simulink model "PhilippePetit"  (R2020b)
settings: Solver=VariableStepAuto  StartTime=0.0  StopTime=10.0  RelTol=1e-3
undefined symbols (not defined in the file or in its folder): den, num_beta, num_x
settings Model: Creator=nicol  LastModifiedBy=nicol

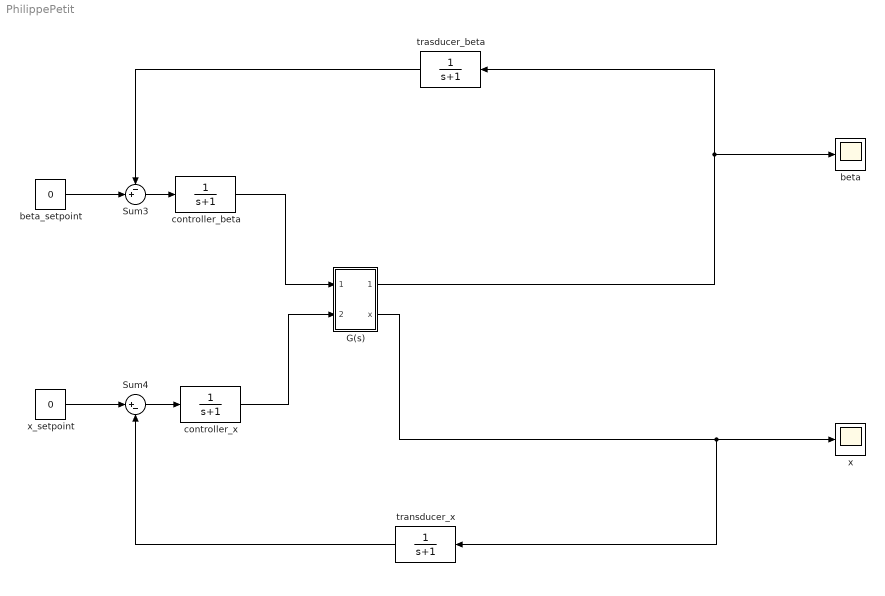
== system PhilippePetit ==
  G(s) : Subsystem
  Sum3 : Sum  Inputs=-+|
  Sum4 : Sum  Inputs=|+-
  beta : Scope
  beta_setpoint : Constant  Value=0
  controller_beta : TransferFcn  Denominator=[1 1]
  controller_x : TransferFcn  Denominator=[1 1]
  transducer_x : TransferFcn  Denominator=[1 1]
  trasducer_beta : TransferFcn  Denominator=[1 1]
  x : Scope
  x_setpoint : Constant  Value=0
  wires:
  trasducer_beta/1 -> Sum3/1
  beta_setpoint/1 -> Sum3/2
  x_setpoint/1 -> Sum4/1
  transducer_x/1 -> Sum4/2
  G(s)/2(x) -> transducer_x/1, x/1
  G(s)/1(beta) -> trasducer_beta/1, beta/1
  Sum3/1 -> controller_beta/1
  Sum4/1 -> controller_x/1
  controller_x/1 -> G(s)/2(In2)
  controller_beta/1 -> G(s)/1(In1)

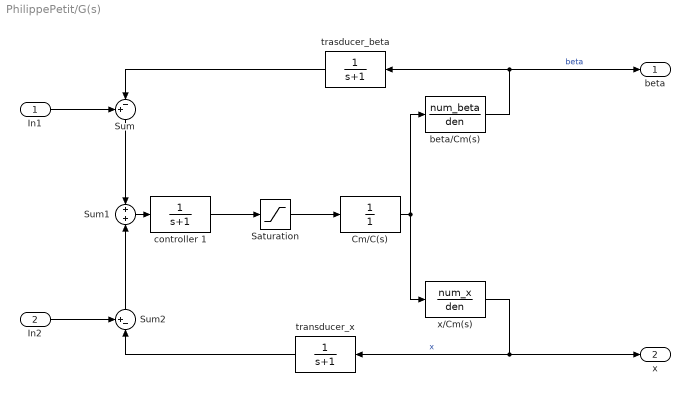
== system PhilippePetit/G(s) ==
  In1 : Inport
  In2 : Inport  Port=2
  Cm/C(s) : TransferFcn  Denominator=[1]
  Saturation : Saturate
  Sum : Sum  Inputs=+-|
  Sum1 : Sum  Inputs=+|+
  Sum2 : Sum  Inputs=+-|
  beta/Cm(s) : TransferFcn  Numerator=num_beta  Denominator=den
  controller 1 : TransferFcn  Denominator=[1 1]
  transducer_x : TransferFcn  Denominator=[1 1]
  trasducer_beta : TransferFcn  Denominator=[1 1]
  x/Cm(s) : TransferFcn  Numerator=num_x  Denominator=den
  beta : Outport
  x : Outport  Port=2
  wires:
  beta/Cm(s)/1 -> trasducer_beta/1, beta/1  "beta"
  Sum/1 -> Sum1/1
  x/Cm(s)/1 -> transducer_x/1, x/1  "x"
  Cm/C(s)/1 -> beta/Cm(s)/1, x/Cm(s)/1
  In1/1 -> Sum/1
  Sum2/1 -> Sum1/2
  Saturation/1 -> Cm/C(s)/1
  Sum1/1 -> controller 1/1
  controller 1/1 -> Saturation/1
  In2/1 -> Sum2/1
  trasducer_beta/1 -> Sum/2
  transducer_x/1 -> Sum2/2
